simulink library "FInjLib"  (R2022b)
settings: Solver=VariableStepAuto  StartTime=0.0  StopTime=10.0  RelTol=1e-3
libraries: simulink x2, $bdroot x2
(part 2 of 2)

== system FInjLib/Negate ==
  note: If fault type == 1 i.e. , Infinite time
      | else fault type == 2 i.e. , constant time,
      | generate correpsonding pulse which is used to enable if-else subsystem
  In1 : Inport
  Constant_to_compare_fault_type : Constant
  Enable_flag : Constant
  Equal : RelationalOperator  Operator===  OutDataTypeStr=boolean  RndMeth=Simplest  InputSameDT=off
  Faulttype : Constant  Value=2
  If : If
  If Action Subsystem : Subsystem  TreatAsAtomicUnit=on
  If Action Subsystem1 : Subsystem  TreatAsAtomicUnit=on
  MainSwitch : Switch  Criteria=u2 > Threshold  SaturateOnIntegerOverflow=off  InputSameDT=off
  Merge : Merge
  Pulse Generator : DiscretePulseGenerator  Period=500  PulseWidth=3  PhaseDelay=2
  Step : Step  Time=4  SampleTime=0
  Switch : Switch  Criteria=u2 > Threshold  SaturateOnIntegerOverflow=off  InputSameDT=off
  Unary Minus : UnaryMinus
  Out1 : Outport  VectorParamsAs1DForOutWhenUnconnected=off
  wires:
  Faulttype/1 -> Equal/1
  Merge/1 -> MainSwitch/1
  If Action Subsystem1/1(Out1) -> Merge/2
  Unary Minus/1 -> If Action Subsystem/1(In1)
  MainSwitch/1 -> Out1/1
  If/1 -> If Action Subsystem/Action
  Step/1 -> Switch/1
  Enable_flag/1 -> MainSwitch/2
  Pulse Generator/1 -> Switch/3
  Constant_to_compare_fault_type/1 -> Equal/2
  If/2 -> If Action Subsystem1/Action
  If Action Subsystem/1(Out1) -> Merge/1
  Equal/1 -> Switch/2
  Switch/1 -> If/1
  In1/1 -> MainSwitch/3, Unary Minus/1, If Action Subsystem1/1(In1)

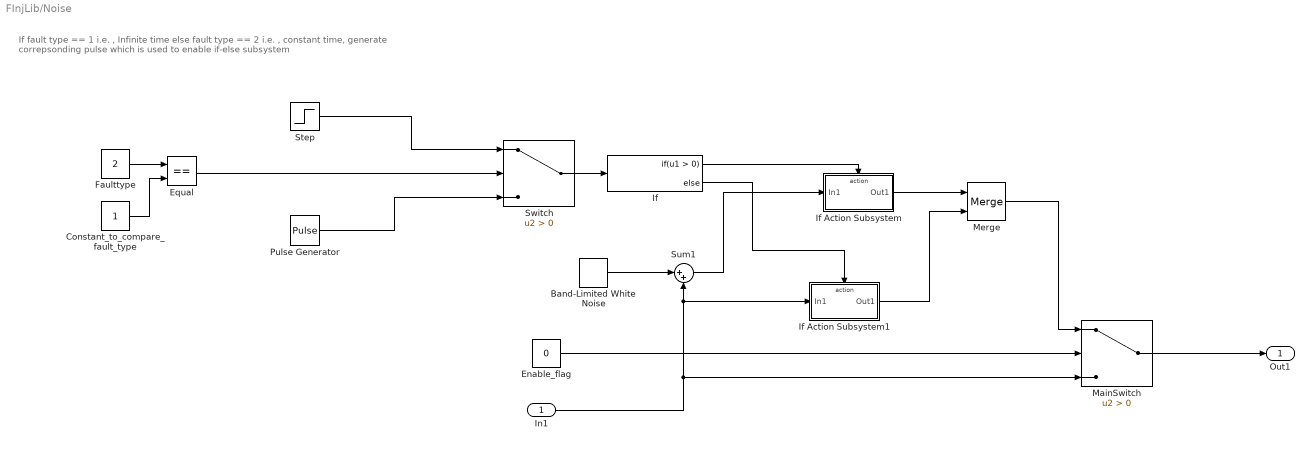
== system FInjLib/Noise ==
  note: If fault type == 1 i.e. , Infinite time
      | else fault type == 2 i.e. , constant time,
      | generate correpsonding pulse which is used to enable if-else subsystem
  In1 : Inport
  Band-Limited White Noise : simulink/Sources/Band-Limited White Noise  Cov=1  Ts=0.04  seed=[23341]
  Constant_to_compare_fault_type : Constant
  Enable_flag : Constant  Value=0
  Equal : RelationalOperator  Operator===  OutDataTypeStr=boolean  RndMeth=Simplest  InputSameDT=off
  Faulttype : Constant  Value=2
  If : If
  If Action Subsystem : Subsystem  TreatAsAtomicUnit=on
  If Action Subsystem1 : Subsystem  TreatAsAtomicUnit=on
  MainSwitch : Switch  Criteria=u2 > Threshold  SaturateOnIntegerOverflow=off  InputSameDT=off
  Merge : Merge
  Pulse Generator : DiscretePulseGenerator  Period=500  PulseWidth=4  PhaseDelay=2
  Step : Step  Time=10  SampleTime=0
  Sum1 : Sum  Inputs=|++
  Switch : Switch  Criteria=u2 > Threshold  SaturateOnIntegerOverflow=off  InputSameDT=off
  Out1 : Outport  VectorParamsAs1DForOutWhenUnconnected=off
  wires:
  Sum1/1 -> If Action Subsystem/1(In1)
  Switch/1 -> If/1
  If Action Subsystem1/1(Out1) -> Merge/2
  Step/1 -> Switch/1
  Equal/1 -> Switch/2
  MainSwitch/1 -> Out1/1
  Faulttype/1 -> Equal/1
  If/1 -> If Action Subsystem/Action
  If/2 -> If Action Subsystem1/Action
  Band-Limited White Noise/1 -> Sum1/1
  Merge/1 -> MainSwitch/1
  In1/1 -> MainSwitch/3, If Action Subsystem1/1(In1), Sum1/2
  Enable_flag/1 -> MainSwitch/2
  Pulse Generator/1 -> Switch/3
  If Action Subsystem/1(Out1) -> Merge/1
  Constant_to_compare_fault_type/1 -> Equal/2

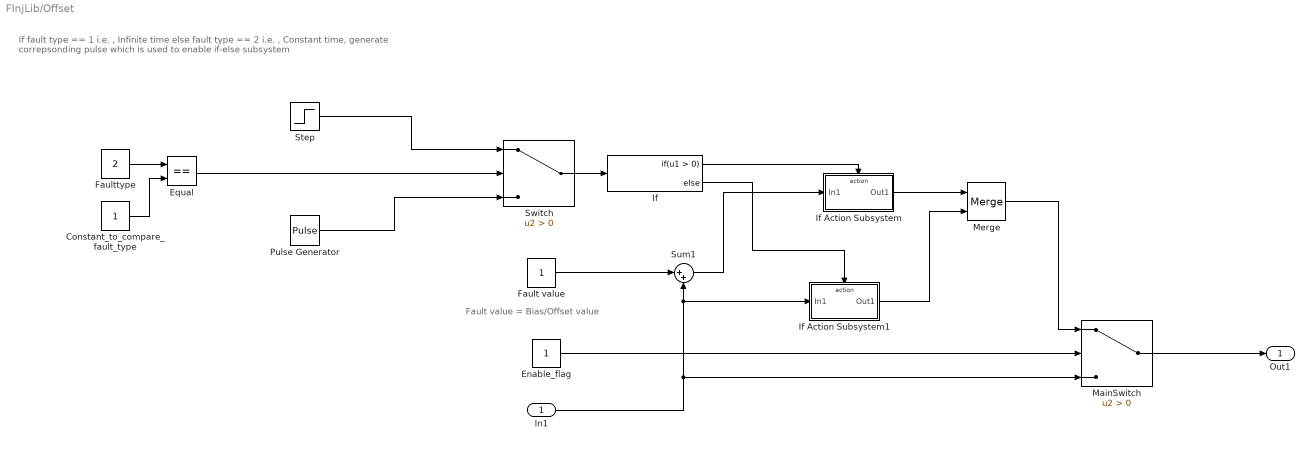
== system FInjLib/Offset ==
  note: If fault type == 1 i.e. , Infinite time
      | else fault type == 2 i.e. , Constant time,
      | generate correpsonding pulse which is used to enable if-else subsystem
  note: Fault value = Bias/Offset value
  In1 : Inport
  Constant_to_compare_fault_type : Constant
  Enable_flag : Constant
  Equal : RelationalOperator  Operator===  OutDataTypeStr=boolean  RndMeth=Simplest  InputSameDT=off
  Fault value : Constant
  Faulttype : Constant  Value=2
  If : If
  If Action Subsystem : Subsystem  TreatAsAtomicUnit=on
  If Action Subsystem1 : Subsystem  TreatAsAtomicUnit=on
  MainSwitch : Switch  Criteria=u2 > Threshold  SaturateOnIntegerOverflow=off  InputSameDT=off
  Merge : Merge
  Pulse Generator : DiscretePulseGenerator  Period=500  PulseWidth=3  PhaseDelay=2
  Step : Step  Time=4  SampleTime=0
  Sum1 : Sum  Inputs=|++
  Switch : Switch  Criteria=u2 > Threshold  SaturateOnIntegerOverflow=off  InputSameDT=off
  Out1 : Outport  VectorParamsAs1DForOutWhenUnconnected=off
  wires:
  If Action Subsystem/1(Out1) -> Merge/1
  Switch/1 -> If/1
  Constant_to_compare_fault_type/1 -> Equal/2
  If/2 -> If Action Subsystem1/Action
  In1/1 -> MainSwitch/3, If Action Subsystem1/1(In1), Sum1/2
  Faulttype/1 -> Equal/1
  Step/1 -> Switch/1
  Merge/1 -> MainSwitch/1
  Pulse Generator/1 -> Switch/3
  Fault value/1 -> Sum1/1
  Sum1/1 -> If Action Subsystem/1(In1)
  If Action Subsystem1/1(Out1) -> Merge/2
  Enable_flag/1 -> MainSwitch/2
  Equal/1 -> Switch/2
  If/1 -> If Action Subsystem/Action
  MainSwitch/1 -> Out1/1

== system FInjLib/PackageDrop ==
  note: If fault type == 1 i.e. , Infinite time
      | else fault type == 2 i.e. , constant time,
      | generate correpsonding pulse which is used to enable if-else subsystem
  In1 : Inport
  Constant_to_compare_fault_type : Constant
  Enable_flag : Constant
  Equal : RelationalOperator  Operator===  OutDataTypeStr=boolean  RndMeth=Simplest  InputSameDT=off
  Fault value : Constant  Value=8
  Faulttype : Constant
  If : If
  If Action Subsystem : $bdroot/Zerofault/If Action Subsystem  SystemSampleTime=-1  VariantActivationTime=update diagram  Latency=0  AutoFrameSizeCalculation=off
  If Action Subsystem1 : $bdroot/Zerofault/If Action Subsystem1  SystemSampleTime=-1  VariantActivationTime=update diagram  Latency=0  AutoFrameSizeCalculation=off
  MainSwitch : Switch  Criteria=u2 > Threshold  SaturateOnIntegerOverflow=off  InputSameDT=off
  Merge : Merge
  Pulse Generator : DiscretePulseGenerator  Period=500  PulseWidth=7  PhaseDelay=6
  Step : Step  Time=6  SampleTime=0
  Switch : Switch  Criteria=u2 > Threshold  SaturateOnIntegerOverflow=off  InputSameDT=off
  Out1 : Outport  VectorParamsAs1DForOutWhenUnconnected=off
  wires:
  Pulse Generator/1 -> Switch/3
  If/1 -> If Action Subsystem/Action
  If Action Subsystem/1 -> Merge/1
  Fault value/1 -> If Action Subsystem/1
  Step/1 -> Switch/1
  Faulttype/1 -> Equal/1
  In1/1 -> MainSwitch/3, If Action Subsystem1/1
  Enable_flag/1 -> MainSwitch/2
  Equal/1 -> Switch/2
  MainSwitch/1 -> Out1/1
  Constant_to_compare_fault_type/1 -> Equal/2
  If/2 -> If Action Subsystem1/Action
  Switch/1 -> If/1
  Merge/1 -> MainSwitch/1
  If Action Subsystem1/1 -> Merge/2

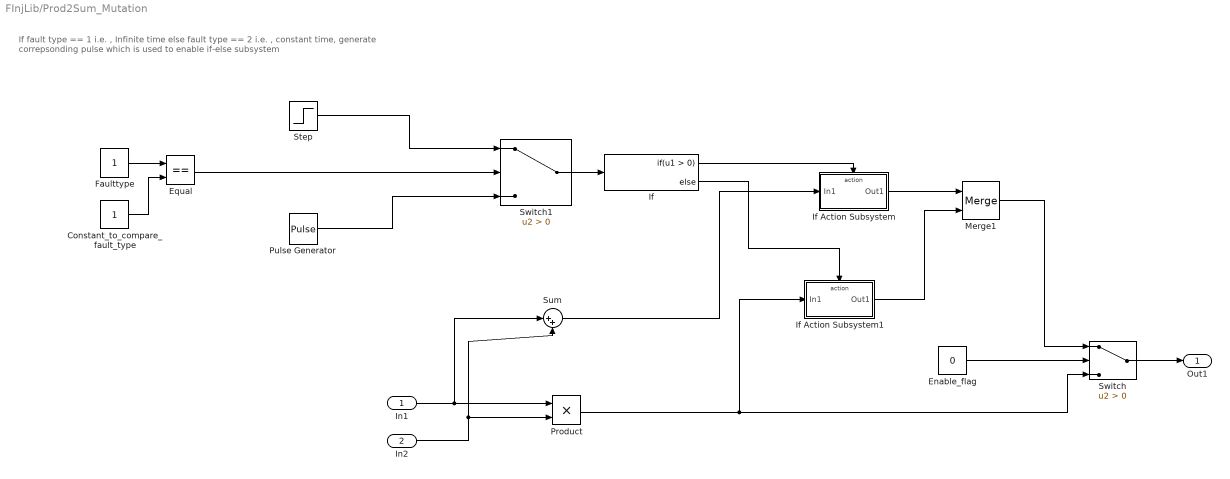
== system FInjLib/Prod2Sum_Mutation ==
  note: If fault type == 1 i.e. , Infinite time
      | else fault type == 2 i.e. , constant time,
      | generate correpsonding pulse which is used to enable if-else subsystem
  In1 : Inport
  In2 : Inport  Port=2
  Constant_to_compare_fault_type : Constant
  Enable_flag : Constant  Value=0
  Equal : RelationalOperator  Operator===  OutDataTypeStr=boolean  RndMeth=Simplest  InputSameDT=off
  Faulttype : Constant
  If : If
  If Action Subsystem : Subsystem  TreatAsAtomicUnit=on
  If Action Subsystem1 : Subsystem  TreatAsAtomicUnit=on
  Merge1 : Merge
  Product : Product
  Pulse Generator : DiscretePulseGenerator  Period=500  PulseWidth=8  PhaseDelay=2
  Step : Step  Time=7  SampleTime=0
  Sum : Sum  Inputs=|++
  Switch : Switch  Criteria=u2 > Threshold  SaturateOnIntegerOverflow=off  InputSameDT=off
  Switch1 : Switch  Criteria=u2 > Threshold  SaturateOnIntegerOverflow=off  InputSameDT=off
  Out1 : Outport  VectorParamsAs1DForOutWhenUnconnected=off
  wires:
  Equal/1 -> Switch1/2
  Sum/1 -> If Action Subsystem/1(In1)
  Product/1 -> If Action Subsystem1/1(In1), Switch/3
  Pulse Generator/1 -> Switch1/3
  Switch/1 -> Out1/1
  If Action Subsystem/1(Out1) -> Merge1/1
  Constant_to_compare_fault_type/1 -> Equal/2
  Faulttype/1 -> Equal/1
  In1/1 -> Sum/1, Product/1
  Step/1 -> Switch1/1
  Switch1/1 -> If/1
  If/1 -> If Action Subsystem/Action
  In2/1 -> Product/2, Sum/2
  If Action Subsystem1/1(Out1) -> Merge1/2
  Merge1/1 -> Switch/1
  Enable_flag/1 -> Switch/2
  If/2 -> If Action Subsystem1/Action

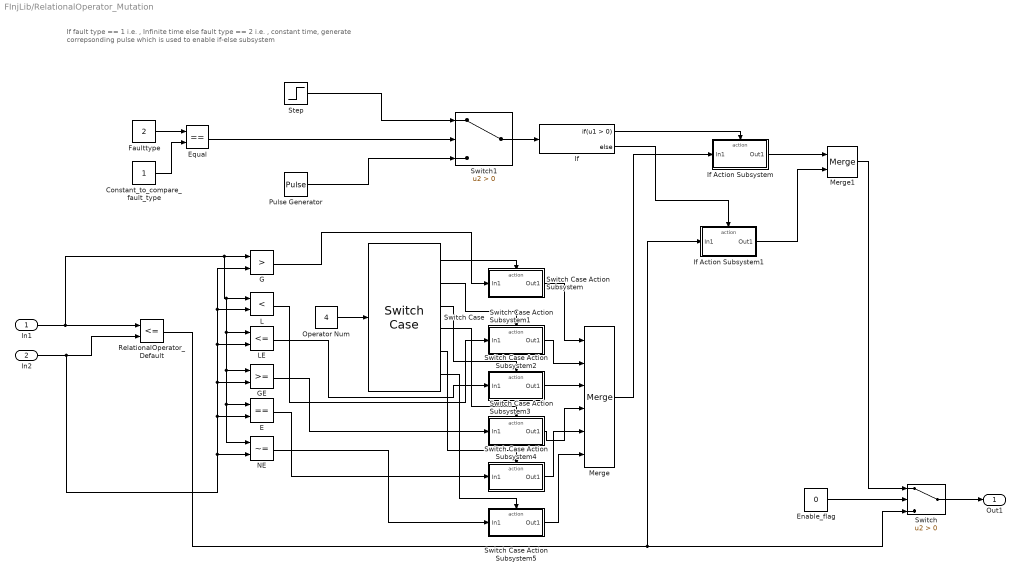
== system FInjLib/RelationalOperator_Mutation ==
  note: If fault type == 1 i.e. , Infinite time
      | else fault type == 2 i.e. , constant time,
      | generate correpsonding pulse which is used to enable if-else subsystem
  In1 : Inport
  In2 : Inport  Port=2
  Constant_to_compare_fault_type : Constant
  E : RelationalOperator  Operator===  OutDataTypeStr=boolean  RndMeth=Simplest  InputSameDT=off
  Enable_flag : Constant  Value=0
  Equal : RelationalOperator  Operator===  OutDataTypeStr=boolean  RndMeth=Simplest  InputSameDT=off
  Faulttype : Constant  Value=2
  "G " : RelationalOperator  Operator=>  OutDataTypeStr=boolean  RndMeth=Simplest  InputSameDT=off
  GE : RelationalOperator  OutDataTypeStr=boolean  RndMeth=Simplest  InputSameDT=off
  If : If
  If Action Subsystem : Subsystem  TreatAsAtomicUnit=on
  If Action Subsystem1 : Subsystem  TreatAsAtomicUnit=on
  L : RelationalOperator  Operator=<  OutDataTypeStr=boolean  RndMeth=Simplest  InputSameDT=off
  LE : RelationalOperator  Operator=<=  OutDataTypeStr=boolean  RndMeth=Simplest  InputSameDT=off
  Merge : Merge  Inputs=6
  Merge1 : Merge
  NE : RelationalOperator  Operator=~=  OutDataTypeStr=boolean  RndMeth=Simplest  InputSameDT=off
  Operator Num : Constant  Value=4
  Pulse Generator : DiscretePulseGenerator  Period=500  PulseWidth=3  PhaseDelay=2
  RelationalOperator_Default : RelationalOperator  Operator=<=  OutDataTypeStr=boolean  RndMeth=Simplest  InputSameDT=off
  Step : Step  Time=5  SampleTime=0
  Switch : Switch  Criteria=u2 > Threshold  SaturateOnIntegerOverflow=off  InputSameDT=off
  Switch Case : SwitchCase  CaseConditions={1,2,3,4,5,6}  ShowDefaultCase=off
  Switch Case Action Subsystem : Subsystem  TreatAsAtomicUnit=on
  Switch Case Action Subsystem1 : Subsystem  TreatAsAtomicUnit=on
  Switch Case Action Subsystem2 : Subsystem  TreatAsAtomicUnit=on
  Switch Case Action Subsystem3 : Subsystem  TreatAsAtomicUnit=on
  Switch Case Action Subsystem4 : Subsystem  TreatAsAtomicUnit=on
  Switch Case Action Subsystem5 : Subsystem  TreatAsAtomicUnit=on
  Switch1 : Switch  Criteria=u2 > Threshold  SaturateOnIntegerOverflow=off  InputSameDT=off
  Out1 : Outport  VectorParamsAs1DForOutWhenUnconnected=off
  wires:
  Switch/1 -> Out1/1
  Switch Case/4 -> Switch Case Action Subsystem3/Action
  If/2 -> If Action Subsystem1/Action
  Switch Case Action Subsystem2/1(Out1) -> Merge/3
  Switch Case/2 -> Switch Case Action Subsystem1/Action
  NE/1 -> Switch Case Action Subsystem5/1(In1)
  Pulse Generator/1 -> Switch1/3
  E/1 -> Switch Case Action Subsystem4/1(In1)
  Switch Case Action Subsystem/1(Out1) -> Merge/1
  Merge1/1 -> Switch/1
  Operator Num/1 -> Switch Case/1
  Switch Case Action Subsystem5/1(Out1) -> Merge/6
  Constant_to_compare_fault_type/1 -> Equal/2
  Switch Case Action Subsystem1/1(Out1) -> Merge/2
  Switch1/1 -> If/1
  Switch Case Action Subsystem3/1(Out1) -> Merge/4
  Enable_flag/1 -> Switch/2
  Switch Case/1 -> Switch Case Action Subsystem/Action
  Faulttype/1 -> Equal/1
  If Action Subsystem1/1(Out1) -> Merge1/2
  GE/1 -> Switch Case Action Subsystem3/1(In1)
  Step/1 -> Switch1/1
  In1/1 -> NE/1, E/1, GE/1, LE/1, L/1, "G "/1, RelationalOperator_Default/1
  "G "/1 -> Switch Case Action Subsystem/1(In1)
  Switch Case Action Subsystem4/1(Out1) -> Merge/5
  RelationalOperator_Default/1 -> Switch/3, If Action Subsystem1/1(In1)
  If Action Subsystem/1(Out1) -> Merge1/1
  L/1 -> Switch Case Action Subsystem1/1(In1)
  Equal/1 -> Switch1/2
  If/1 -> If Action Subsystem/Action
  LE/1 -> Switch Case Action Subsystem2/1(In1)
  In2/1 -> E/2, LE/2, L/2, "G "/2, GE/2, NE/2, RelationalOperator_Default/2
  Merge/1 -> If Action Subsystem/1(In1)
  Switch Case/3 -> Switch Case Action Subsystem2/Action
  Switch Case/5 -> Switch Case Action Subsystem4/Action
  Switch Case/6 -> Switch Case Action Subsystem5/Action

== system FInjLib/Stuck-at ==
  note: If fault type == 1 i.e. , Infinite time
      | else fault type == 2 i.e. , constant time,
      | generate correpsonding pulse which is used to enable if-else subsystem
  In1 : Inport
  Constant_to_compare_fault_type : Constant
  Enable_flag : Constant
  Equal : RelationalOperator  Operator===  OutDataTypeStr=boolean  RndMeth=Simplest  InputSameDT=off
  Faulttype : Constant
  MainSwitch : Switch  Criteria=u2 > Threshold  SaturateOnIntegerOverflow=off  InputSameDT=off
  MainSwitch1 : Switch  Criteria=u2 > Threshold  SaturateOnIntegerOverflow=off  InputSameDT=off
  Memory : Memory  InheritSampleTime=on
  NOT : Logic  Operator=NOT  IconShape=distinctive  AllPortsSameDT=off  OutDataTypeStr=boolean
  Pulse Generator : DiscretePulseGenerator  Period=500  PulseWidth=6  PhaseDelay=4
  Step : Step  Time=4  SampleTime=0
  Switch : Switch  Criteria=u2 > Threshold  SaturateOnIntegerOverflow=off  InputSameDT=off
  Out1 : Outport  VectorParamsAs1DForOutWhenUnconnected=off
  wires:
  Equal/1 -> Switch/2
  In1/1 -> MainSwitch1/1, MainSwitch/3
  Constant_to_compare_fault_type/1 -> Equal/2
  MainSwitch1/1 -> MainSwitch/1, Memory/1
  Switch/1 -> NOT/1
  NOT/1 -> MainSwitch1/2
  Faulttype/1 -> Equal/1
  Step/1 -> Switch/1
  MainSwitch/1 -> Out1/1
  Pulse Generator/1 -> Switch/3
  Enable_flag/1 -> MainSwitch/2
  Memory/1 -> MainSwitch1/3

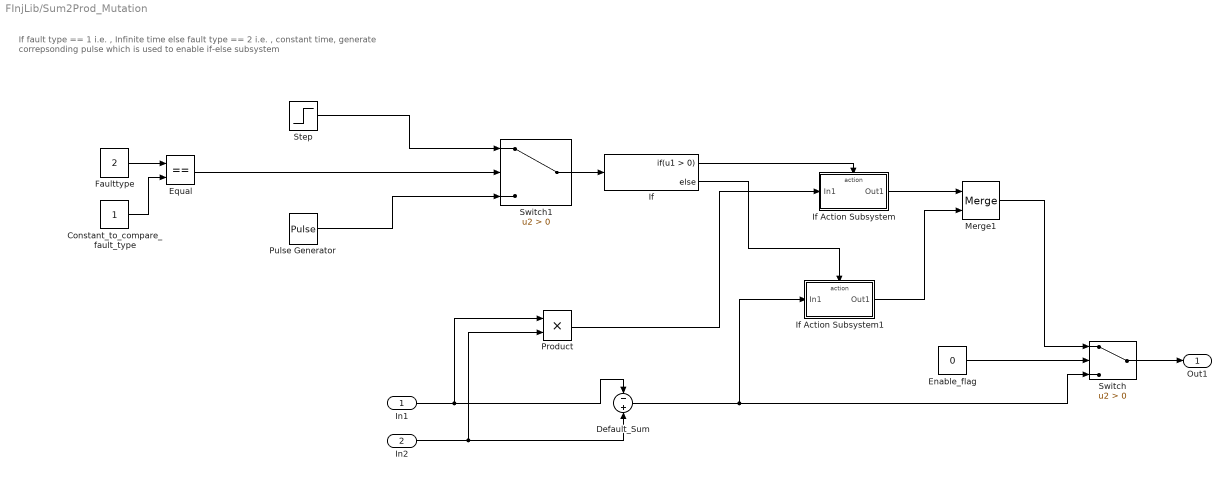
== system FInjLib/Sum2Prod_Mutation ==
  note: If fault type == 1 i.e. , Infinite time
      | else fault type == 2 i.e. , constant time,
      | generate correpsonding pulse which is used to enable if-else subsystem
  In1 : Inport
  In2 : Inport  Port=2
  Constant_to_compare_fault_type : Constant
  Default_Sum : Sum  Inputs=-+
  Enable_flag : Constant  Value=0
  Equal : RelationalOperator  Operator===  OutDataTypeStr=boolean  RndMeth=Simplest  InputSameDT=off
  Faulttype : Constant  Value=2
  If : If
  If Action Subsystem : Subsystem  TreatAsAtomicUnit=on
  If Action Subsystem1 : Subsystem  TreatAsAtomicUnit=on
  Merge1 : Merge
  Product : Product
  Pulse Generator : DiscretePulseGenerator  Period=500  PulseWidth=3  PhaseDelay=5
  Step : Step  Time=8  SampleTime=0
  Switch : Switch  Criteria=u2 > Threshold  SaturateOnIntegerOverflow=off  InputSameDT=off
  Switch1 : Switch  Criteria=u2 > Threshold  SaturateOnIntegerOverflow=off  InputSameDT=off
  Out1 : Outport  VectorParamsAs1DForOutWhenUnconnected=off
  wires:
  Merge1/1 -> Switch/1
  In2/1 -> Product/2, Default_Sum/2
  If Action Subsystem1/1(Out1) -> Merge1/2
  Switch1/1 -> If/1
  Product/1 -> If Action Subsystem/1(In1)
  Default_Sum/1 -> If Action Subsystem1/1(In1), Switch/3
  Constant_to_compare_fault_type/1 -> Equal/2
  If Action Subsystem/1(Out1) -> Merge1/1
  Switch/1 -> Out1/1
  Equal/1 -> Switch1/2
  Enable_flag/1 -> Switch/2
  Pulse Generator/1 -> Switch1/3
  In1/1 -> Product/1, Default_Sum/1
  If/2 -> If Action Subsystem1/Action
  Step/1 -> Switch1/1
  Faulttype/1 -> Equal/1
  If/1 -> If Action Subsystem/Action

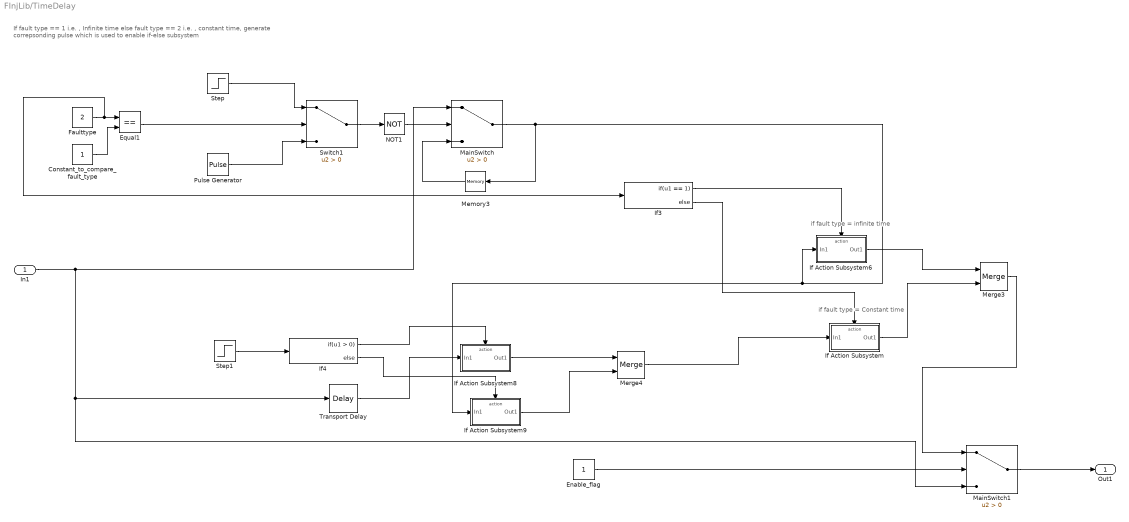
== system FInjLib/TimeDelay ==
  note: If fault type == 1 i.e. , Infinite time
      | else fault type == 2 i.e. , constant time,
      | generate correpsonding pulse which is used to enable if-else subsystem
  note: if fault type = Constant time
  note: if fault type = infinite time
  In1 : Inport
  Constant_to_compare_fault_type : Constant
  Enable_flag : Constant
  Equal1 : RelationalOperator  Operator===  OutDataTypeStr=boolean  RndMeth=Simplest  InputSameDT=off
  Faulttype : Constant  Value=2
  If Action Subsystem : Subsystem  TreatAsAtomicUnit=on
  If Action Subsystem6 : Subsystem  TreatAsAtomicUnit=on
  If Action Subsystem8 : Subsystem  TreatAsAtomicUnit=on
  If Action Subsystem9 : Subsystem  TreatAsAtomicUnit=on
  If3 : If  IfExpression=u1 == 1
  If4 : If
  MainSwitch : Switch  Criteria=u2 > Threshold  SaturateOnIntegerOverflow=off  InputSameDT=off
  MainSwitch1 : Switch  Criteria=u2 > Threshold  SaturateOnIntegerOverflow=off  InputSameDT=off
  Memory3 : Memory  InheritSampleTime=on
  Merge3 : Merge
  Merge4 : Merge
  NOT1 : Logic  Operator=NOT  IconShape=distinctive  AllPortsSameDT=off  OutDataTypeStr=boolean
  Pulse Generator : DiscretePulseGenerator  Period=500  PulseWidth=10  PhaseDelay=10
  Step : Step  Time=4  SampleTime=0
  Step1 : Step  Time=20  SampleTime=0
  Switch1 : Switch  Criteria=u2 > Threshold  SaturateOnIntegerOverflow=off  InputSameDT=off
  Transport Delay : TransportDelay  DelayTime=10
  Out1 : Outport  VectorParamsAs1DForOutWhenUnconnected=off
  wires:
  Constant_to_compare_fault_type/1 -> Equal1/2
  If4/1 -> If Action Subsystem8/Action
  Step/1 -> Switch1/1
  If Action Subsystem8/1(Out1) -> Merge4/1
  If Action Subsystem/1(Out1) -> Merge3/2
  If4/2 -> If Action Subsystem9/Action
  Transport Delay/1 -> If Action Subsystem8/1(In1)
  Merge4/1 -> If Action Subsystem/1(In1)
  Pulse Generator/1 -> Switch1/3
  Step1/1 -> If4/1
  Faulttype/1 -> If3/1, Equal1/1
  If Action Subsystem9/1(Out1) -> Merge4/2
  Memory3/1 -> MainSwitch/3
  Switch1/1 -> NOT1/1
  If Action Subsystem6/1(Out1) -> Merge3/1
  If3/1 -> If Action Subsystem6/Action
  In1/1 -> MainSwitch1/3, Transport Delay/1, MainSwitch/1
  Equal1/1 -> Switch1/2
  If3/2 -> If Action Subsystem/Action
  MainSwitch/1 -> Memory3/1, If Action Subsystem9/1(In1), If Action Subsystem6/1(In1)
  NOT1/1 -> MainSwitch/2
  Enable_flag/1 -> MainSwitch1/2
  MainSwitch1/1 -> Out1/1
  Merge3/1 -> MainSwitch1/1

== system FInjLib/Zerofault ==
  note: If fault type == 1 i.e. , Infinite time
      | else fault type == 2 i.e. , constant time,
      | generate correpsonding pulse which is used to enable if-else subsystem
  In1 : Inport
  Constant_to_compare_fault_type : Constant
  Enable_flag : Constant
  Equal : RelationalOperator  Operator===  OutDataTypeStr=boolean  RndMeth=Simplest  InputSameDT=off
  Faulttype : Constant  Value=2
  If : If
  If Action Subsystem : Subsystem  TreatAsAtomicUnit=on
  If Action Subsystem1 : Subsystem  TreatAsAtomicUnit=on
  MainSwitch : Switch  Criteria=u2 > Threshold  SaturateOnIntegerOverflow=off  InputSameDT=off
  Merge : Merge
  Pulse Generator : DiscretePulseGenerator  Period=500  PulseWidth=10  PhaseDelay=10
  Step : Step  Time=7  SampleTime=0
  Switch : Switch  Criteria=u2 > Threshold  SaturateOnIntegerOverflow=off  InputSameDT=off
  Zero (Constant) : Constant  Value=0
  Out1 : Outport  VectorParamsAs1DForOutWhenUnconnected=off
  wires:
  MainSwitch/1 -> Out1/1
  If Action Subsystem/1(Out1) -> Merge/1
  Constant_to_compare_fault_type/1 -> Equal/2
  Zero (Constant)/1 -> If Action Subsystem/1(In1)
  Faulttype/1 -> Equal/1
  Switch/1 -> If/1
  Pulse Generator/1 -> Switch/3
  Step/1 -> Switch/1
  If Action Subsystem1/1(Out1) -> Merge/2
  Equal/1 -> Switch/2
  If/2 -> If Action Subsystem1/Action
  In1/1 -> MainSwitch/3, If Action Subsystem1/1(In1)
  Merge/1 -> MainSwitch/1
  Enable_flag/1 -> MainSwitch/2
  If/1 -> If Action Subsystem/Action

== system FInjLib/Absolute/If Action Subsystem ==
  In1 : Inport
  Action Port : ActionPort  ActionPortLabel=if { }
  Out1 : Outport  VectorParamsAs1DForOutWhenUnconnected=off
  wires:
  In1/1 -> Out1/1

== system FInjLib/Absolute/If Action Subsystem1 ==
  In1 : Inport
  Action Port : ActionPort  ActionPortLabel=else { }
  Out1 : Outport  VectorParamsAs1DForOutWhenUnconnected=off
  wires:
  In1/1 -> Out1/1

== system FInjLib/ArSignReplOperator/If Action Subsystem ==
  In1 : Inport
  Action Port : ActionPort  ActionPortLabel=if { }
  Out1 : Outport  VectorParamsAs1DForOutWhenUnconnected=off
  wires:
  In1/1 -> Out1/1

== system FInjLib/ArSignReplOperator/If Action Subsystem1 ==
  In1 : Inport
  Action Port : ActionPort  ActionPortLabel=else { }
  Out1 : Outport  VectorParamsAs1DForOutWhenUnconnected=off
  wires:
  In1/1 -> Out1/1

== system FInjLib/ArSignReplOperator/Switch Case Action Subsystem ==
  In1 : Inport
  Action Port : ActionPort  ActionPortLabel=case: { }
  Out1 : Outport  VectorParamsAs1DForOutWhenUnconnected=off
  wires:
  In1/1 -> Out1/1

== system FInjLib/ArSignReplOperator/Switch Case Action Subsystem1 ==
  In1 : Inport
  Action Port : ActionPort  ActionPortLabel=case: { }
  Out1 : Outport  VectorParamsAs1DForOutWhenUnconnected=off
  wires:
  In1/1 -> Out1/1

== system FInjLib/ArSignReplOperator/Switch Case Action Subsystem2 ==
  In1 : Inport
  Action Port : ActionPort  ActionPortLabel=case: { }
  Out1 : Outport  VectorParamsAs1DForOutWhenUnconnected=off
  wires:
  In1/1 -> Out1/1

== system FInjLib/ArSignReplOperator/Switch Case Action Subsystem3 ==
  In1 : Inport
  Action Port : ActionPort  ActionPortLabel=case: { }
  Out1 : Outport  VectorParamsAs1DForOutWhenUnconnected=off
  wires:
  In1/1 -> Out1/1

== system FInjLib/BitFlip/If Action Subsystem ==
  In1 : Inport
  Action Port : ActionPort  ActionPortLabel=if { }
  Out1 : Outport  VectorParamsAs1DForOutWhenUnconnected=off
  wires:
  In1/1 -> Out1/1

== system FInjLib/BitFlip/If Action Subsystem1 ==
  In1 : Inport
  Action Port : ActionPort  ActionPortLabel=else { }
  Out1 : Outport  VectorParamsAs1DForOutWhenUnconnected=off
  wires:
  In1/1 -> Out1/1

== system FInjLib/Inverter/If Action Subsystem ==
  In1 : Inport
  Action Port : ActionPort  ActionPortLabel=if { }
  Out1 : Outport  VectorParamsAs1DForOutWhenUnconnected=off
  wires:
  In1/1 -> Out1/1

== system FInjLib/Inverter/If Action Subsystem1 ==
  In1 : Inport
  Action Port : ActionPort  ActionPortLabel=else { }
  Out1 : Outport  VectorParamsAs1DForOutWhenUnconnected=off
  wires:
  In1/1 -> Out1/1

== system FInjLib/LogicalOperator_Mutation/If Action Subsystem ==
  In1 : Inport
  Action Port : ActionPort  ActionPortLabel=if { }
  Out1 : Outport  VectorParamsAs1DForOutWhenUnconnected=off
  wires:
  In1/1 -> Out1/1

== system FInjLib/LogicalOperator_Mutation/If Action Subsystem1 ==
  In1 : Inport
  Action Port : ActionPort  ActionPortLabel=else { }
  Out1 : Outport  VectorParamsAs1DForOutWhenUnconnected=off
  wires:
  In1/1 -> Out1/1

== system FInjLib/LogicalOperator_Mutation/Switch Case Action Subsystem ==
  In1 : Inport
  Action Port : ActionPort  ActionPortLabel=case: { }
  Out1 : Outport  VectorParamsAs1DForOutWhenUnconnected=off
  wires:
  In1/1 -> Out1/1

== system FInjLib/LogicalOperator_Mutation/Switch Case Action Subsystem1 ==
  In1 : Inport
  Action Port : ActionPort  ActionPortLabel=case: { }
  Out1 : Outport  VectorParamsAs1DForOutWhenUnconnected=off
  wires:
  In1/1 -> Out1/1

== system FInjLib/LogicalOperator_Mutation/Switch Case Action Subsystem2 ==
  In1 : Inport
  Action Port : ActionPort  ActionPortLabel=case: { }
  Out1 : Outport  VectorParamsAs1DForOutWhenUnconnected=off
  wires:
  In1/1 -> Out1/1

== system FInjLib/LogicalOperator_Mutation/Switch Case Action Subsystem3 ==
  In1 : Inport
  Action Port : ActionPort  ActionPortLabel=case: { }
  Out1 : Outport  VectorParamsAs1DForOutWhenUnconnected=off
  wires:
  In1/1 -> Out1/1

== system FInjLib/LogicalOperator_Mutation/Switch Case Action Subsystem4 ==
  In1 : Inport
  Action Port : ActionPort  ActionPortLabel=case: { }
  Out1 : Outport  VectorParamsAs1DForOutWhenUnconnected=off
  wires:
  In1/1 -> Out1/1

== system FInjLib/LogicalOperator_Mutation/Switch Case Action Subsystem5 ==
  In1 : Inport
  Action Port : ActionPort  ActionPortLabel=case: { }
  Out1 : Outport  VectorParamsAs1DForOutWhenUnconnected=off
  wires:
  In1/1 -> Out1/1

== system FInjLib/Negate/If Action Subsystem ==
  In1 : Inport
  Action Port : ActionPort
  Out1 : Outport  VectorParamsAs1DForOutWhenUnconnected=off
  wires:
  In1/1 -> Out1/1

== system FInjLib/Negate/If Action Subsystem1 ==
  In1 : Inport
  Action Port : ActionPort
  Out1 : Outport  VectorParamsAs1DForOutWhenUnconnected=off
  wires:
  In1/1 -> Out1/1

== system FInjLib/Noise/If Action Subsystem ==
  In1 : Inport
  Action Port : ActionPort  ActionPortLabel=if { }
  Out1 : Outport  VectorParamsAs1DForOutWhenUnconnected=off
  wires:
  In1/1 -> Out1/1

== system FInjLib/Noise/If Action Subsystem1 ==
  In1 : Inport
  Action Port : ActionPort  ActionPortLabel=else { }
  Out1 : Outport  VectorParamsAs1DForOutWhenUnconnected=off
  wires:
  In1/1 -> Out1/1

== system FInjLib/Offset/If Action Subsystem ==
  In1 : Inport
  Action Port : ActionPort
  Out1 : Outport  VectorParamsAs1DForOutWhenUnconnected=off
  wires:
  In1/1 -> Out1/1

== system FInjLib/Offset/If Action Subsystem1 ==
  In1 : Inport
  Action Port : ActionPort
  Out1 : Outport  VectorParamsAs1DForOutWhenUnconnected=off
  wires:
  In1/1 -> Out1/1

== system FInjLib/Prod2Sum_Mutation/If Action Subsystem ==
  In1 : Inport
  Action Port : ActionPort
  Out1 : Outport  VectorParamsAs1DForOutWhenUnconnected=off
  wires:
  In1/1 -> Out1/1

== system FInjLib/Prod2Sum_Mutation/If Action Subsystem1 ==
  In1 : Inport
  Action Port : ActionPort
  Out1 : Outport  VectorParamsAs1DForOutWhenUnconnected=off
  wires:
  In1/1 -> Out1/1

== system FInjLib/RelationalOperator_Mutation/If Action Subsystem ==
  In1 : Inport
  Action Port : ActionPort  ActionPortLabel=if { }
  Out1 : Outport  VectorParamsAs1DForOutWhenUnconnected=off
  wires:
  In1/1 -> Out1/1

== system FInjLib/RelationalOperator_Mutation/If Action Subsystem1 ==
  In1 : Inport
  Action Port : ActionPort  ActionPortLabel=else { }
  Out1 : Outport  VectorParamsAs1DForOutWhenUnconnected=off
  wires:
  In1/1 -> Out1/1

== system FInjLib/RelationalOperator_Mutation/Switch Case Action Subsystem ==
  In1 : Inport
  Action Port : ActionPort  ActionPortLabel=case: { }
  Out1 : Outport  VectorParamsAs1DForOutWhenUnconnected=off
  wires:
  In1/1 -> Out1/1

== system FInjLib/RelationalOperator_Mutation/Switch Case Action Subsystem1 ==
  In1 : Inport
  Action Port : ActionPort  ActionPortLabel=case: { }
  Out1 : Outport  VectorParamsAs1DForOutWhenUnconnected=off
  wires:
  In1/1 -> Out1/1

== system FInjLib/RelationalOperator_Mutation/Switch Case Action Subsystem2 ==
  In1 : Inport
  Action Port : ActionPort  ActionPortLabel=case: { }
  Out1 : Outport  VectorParamsAs1DForOutWhenUnconnected=off
  wires:
  In1/1 -> Out1/1

== system FInjLib/RelationalOperator_Mutation/Switch Case Action Subsystem3 ==
  In1 : Inport
  Action Port : ActionPort  ActionPortLabel=case: { }
  Out1 : Outport  VectorParamsAs1DForOutWhenUnconnected=off
  wires:
  In1/1 -> Out1/1

== system FInjLib/RelationalOperator_Mutation/Switch Case Action Subsystem4 ==
  In1 : Inport
  Action Port : ActionPort  ActionPortLabel=case: { }
  Out1 : Outport  VectorParamsAs1DForOutWhenUnconnected=off
  wires:
  In1/1 -> Out1/1

== system FInjLib/RelationalOperator_Mutation/Switch Case Action Subsystem5 ==
  In1 : Inport
  Action Port : ActionPort  ActionPortLabel=case: { }
  Out1 : Outport  VectorParamsAs1DForOutWhenUnconnected=off
  wires:
  In1/1 -> Out1/1

== system FInjLib/Sum2Prod_Mutation/If Action Subsystem ==
  In1 : Inport
  Action Port : ActionPort  ActionPortLabel=if { }
  Out1 : Outport  VectorParamsAs1DForOutWhenUnconnected=off
  wires:
  In1/1 -> Out1/1

== system FInjLib/Sum2Prod_Mutation/If Action Subsystem1 ==
  In1 : Inport
  Action Port : ActionPort  ActionPortLabel=else { }
  Out1 : Outport  VectorParamsAs1DForOutWhenUnconnected=off
  wires:
  In1/1 -> Out1/1

== system FInjLib/TimeDelay/If Action Subsystem ==
  In1 : Inport
  Action Port : ActionPort  ActionPortLabel=else { }
  Out1 : Outport  VectorParamsAs1DForOutWhenUnconnected=off
  wires:
  In1/1 -> Out1/1

== system FInjLib/TimeDelay/If Action Subsystem6 ==
  In1 : Inport
  Action Port : ActionPort  ActionPortLabel=if { }
  Out1 : Outport  VectorParamsAs1DForOutWhenUnconnected=off
  wires:
  In1/1 -> Out1/1

== system FInjLib/TimeDelay/If Action Subsystem8 ==
  In1 : Inport
  Action Port : ActionPort  ActionPortLabel=if { }
  Out1 : Outport  VectorParamsAs1DForOutWhenUnconnected=off
  wires:
  In1/1 -> Out1/1

== system FInjLib/TimeDelay/If Action Subsystem9 ==
  In1 : Inport
  Action Port : ActionPort  ActionPortLabel=else { }
  Out1 : Outport  VectorParamsAs1DForOutWhenUnconnected=off
  wires:
  In1/1 -> Out1/1

== system FInjLib/Zerofault/If Action Subsystem ==
  In1 : Inport
  Action Port : ActionPort  ActionPortLabel=if { }
  Out1 : Outport  VectorParamsAs1DForOutWhenUnconnected=off
  wires:
  In1/1 -> Out1/1

== system FInjLib/Zerofault/If Action Subsystem1 ==
  In1 : Inport
  Action Port : ActionPort  ActionPortLabel=else { }
  Out1 : Outport  VectorParamsAs1DForOutWhenUnconnected=off
  wires:
  In1/1 -> Out1/1
